simulink model "Ingenuo1Simulink"  (R2022b)
settings: Solver=VariableStepAuto  StartTime=0.0  StopTime=10.0  RelTol=1e-3
libraries: cstblocks x2
settings Model: Creator=Ares-  LastModifiedBy=Ares-

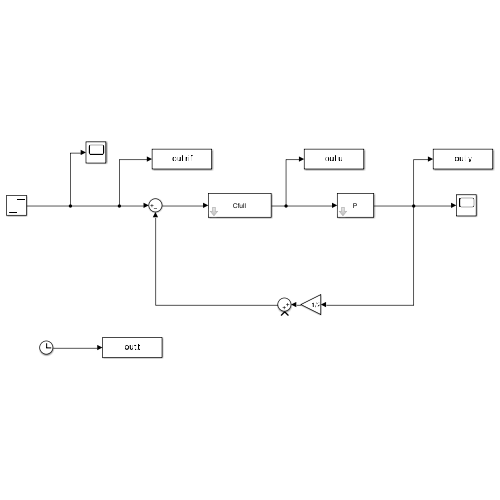
[thumbnail: Simulink's stored preview of the top-level diagram]
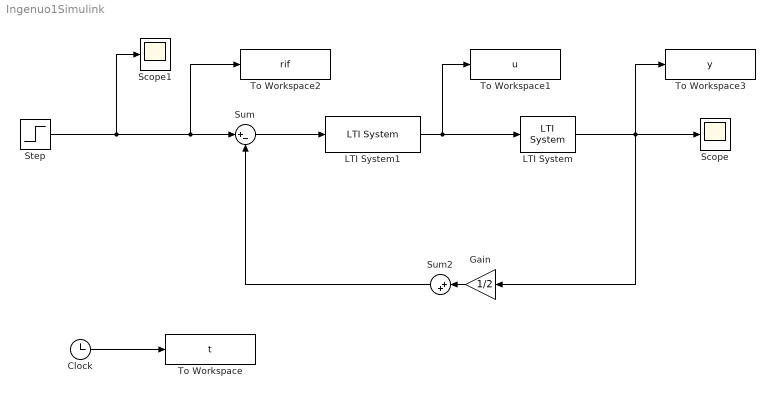
== system Ingenuo1Simulink ==
  Clock : Clock
  Gain : Gain  Gain=1/2
  LTI System : cstblocks/LTI System  sys=P  IC=[]
  LTI System1 : cstblocks/LTI System  sys=Cfull  IC=[]
  Scope : Scope
  Scope1 : Scope
  Step : Step  Time=0  SampleTime=0
  Sum : Sum  Inputs=|+-
  Sum2 : Sum  Inputs=|++
  To Workspace : ToWorkspace  VariableName=t  SampleTime=-1
  To Workspace1 : ToWorkspace  VariableName=u  SampleTime=-1
  To Workspace2 : ToWorkspace  VariableName=rif  SampleTime=-1
  To Workspace3 : ToWorkspace  VariableName=y  SampleTime=-1
  wires:
  Step/1 -> To Workspace2/1, Sum/1, Scope1/1
  Sum2/1 -> Sum/2
  Gain/1 -> Sum2/1
  LTI System/1 -> To Workspace3/1, Scope/1, Gain/1
  LTI System1/1 -> LTI System/1, To Workspace1/1
  Sum/1 -> LTI System1/1
  Clock/1 -> To Workspace/1
